simulink model "launchpad"  (R2014a)
settings: Solver=FixedStepDiscrete  StartTime=0.0  StopTime=10  FixedStep=0.1  RelTol=1e-3
PreLoadFcn:
  | use_hardware = 0;
  | hardware_variant = Simulink.Variant('use_hardware == 1');
  | software_variant = Simulink.Variant('use_hardware == 0');
undefined symbols (not defined in the file or in its folder): sigbuilder_block
libraries: launchpad_lib x5, simulink x1
settings Model: Creator=bas  LastModifiedBy=peselnikmg
settings OptimizationCC: InlineParams=on  UseFloatMulNetSlope=on  UseSpecifiedMinMax=on  InlineInvariantSignals=on  ExpressionDepthLimit=2147483647  ZeroExternalMemoryAtStartup=off  ZeroInternalMemoryAtStartup=off  NoFixptDivByZeroProtection=on  EfficientFloat2IntCast=on  OptimizeModelRefInitCode=on  LifeSpan=Inf
settings DebuggingCC: MergeDetectMultiDrivingBlocksExec=error  InheritedTsInSrcMsg=none  StateNameClashWarn=warning  StrictBusMsg=ErrorOnBusTreatedAsVector
settings HardwareCC: ProdBitPerInt=16  ProdBitPerPointer=16  ProdIntDivRoundTo=Zero  ProdEndianess=LittleEndian  ProdWordSize=16  ProdHWDeviceType=Texas Instruments->MSP430
settings RTWCC: SystemTargetFile=launchpad.tlc  TemplateMakefile=launchpad_tmf  Description=TI LaunchPad  GenerateReport=on  ProcessScript=launchpad_make_rtw_hook  IncludeHyperlinkInReport=on  LaunchReport=on  GenerateTraceInfo=on  GenerateTraceReport=on  GenerateTraceReportSl=on  GenerateTraceReportSf=on  GenerateTraceReportEml=on  GenerateCodeMetricsReport=on
settings CodeAppCC: IgnoreCustomStorageClasses=off  CustomSymbolStrType=$N$R$M  InternalIdentifier=Classic
settings STFCustomTargetCC: ConcurrentExecutionCompliant=off  IncludeMdlTerminateFcn=off  GeneratePreprocessorConditionals=Use local settings  CombineOutputUpdateFcns=on  CombineSignalStateStructs=on  SuppressErrorStatus=on  ERTCustomFileBanners=on  SupportNonFinite=off  SupportContinuousTime=off  SupportNonInlinedSFcns=off  MATLABClassNameForMDSCustomization=Simulink.SoftwareTarget.ERTCustomization  GRTInterface=off  SystemTargetFile=launchpad.tlc
settings ERTTargetCC: GenerateSampleERTMain=off  IncludeMdlTerminateFcn=off  CombineSignalStateStructs=on  SuppressErrorStatus=on  SupportNonFinite=off  ExtModeMexFile=noextcomm  ERTCustomFileTemplate=launchpad_srmain.tlc  ConvertIfToSwitch=on  SuppressUnreachableDefaultCases=on

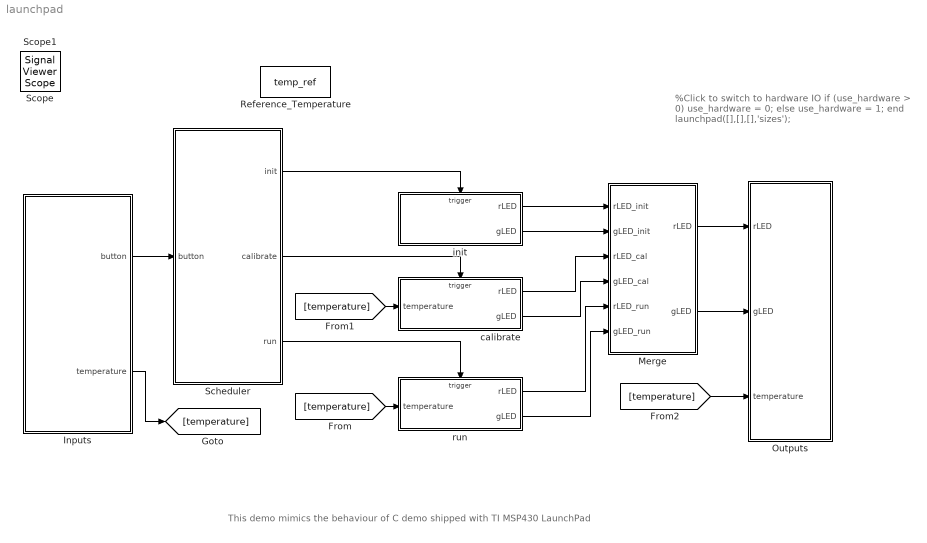
== system launchpad ==
  note: This demo mimics the behaviour of C demo shipped with TI MSP430 LaunchPad
  note: %Click to switch to hardware IO
      | if (use_hardware > 0)
      |     use_hardware = 0;
      | else
      |     use_hardware = 1;
      | end
      | launchpad([],[],[],'sizes');
  Inputs : Subsystem  Variant=on
  Merge : Subsystem
  Outputs : Subsystem  Variant=on
  Reference_Temperature : DataStoreMemory  DataStoreName=temp_ref  ReadBeforeWriteMsg=warning  WriteAfterWriteMsg=warning  WriteAfterReadMsg=warning  OutDataTypeStr=int8
  Scheduler : Subsystem
  calibrate : Subsystem
  init : Subsystem
  run : Subsystem
  Scope : SignalViewerScope  IOType=viewer  NumInputPorts=3  RefreshTime=0.035000
      settings: TimeRange=10  YMin=0~0~0  YMax=1~120~1
  Scope1 : SignalViewerScope  IOType=viewer  RefreshTime=0.035000
  wires:
  Scheduler/2(calibrate) -> calibrate/Trigger
  Scheduler/3(run) -> run/Trigger
  Inputs/1(button) -> Scheduler/1(button)
  Merge/1(rLED) -> Outputs/1(rLED)
  Merge/2(gLED) -> Outputs/2(gLED)
  calibrate/1(rLED) -> Merge/3(rLED_cal)
  calibrate/2(gLED) -> Merge/4(gLED_cal)
  run/1(rLED) -> Merge/5(rLED_run)
  run/2(gLED) -> Merge/6(gLED_run)
  init/1(rLED) -> Merge/1(rLED_init)
  init/2(gLED) -> Merge/2(gLED_init)
  Inputs/2(temperature) -> [temperature]
  [temperature] -> run/1(temperature)
  [temperature] -> calibrate/1(temperature)
  [temperature] -> Outputs/3(temperature)
  Scheduler/1(init) -> init/Trigger

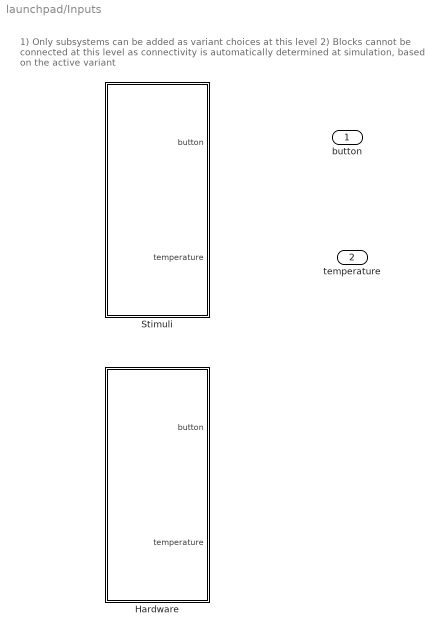
== system launchpad/Inputs ==
  note: 1) Only subsystems can be added as variant choices at this level
      | 2) Blocks cannot be connected at this level as connectivity is
      | automatically determined at simulation, based on the active variant
  Hardware : Subsystem  VariantControl=hardware_variant
  Stimuli : Subsystem  VariantControl=software_variant
  button : Outport
  temperature : Outport  Port=2

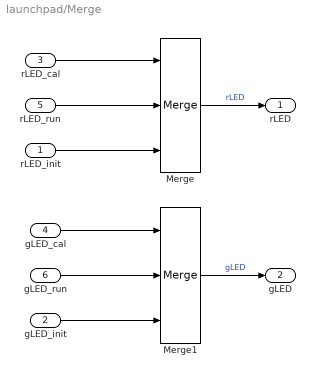
== system launchpad/Merge ==
  rLED_init : Inport
  gLED_init : Inport  Port=2
  rLED_cal : Inport  Port=3
  gLED_cal : Inport  Port=4
  rLED_run : Inport  Port=5
  gLED_run : Inport  Port=6
  Merge : Merge  Inputs=3  InitialOutput=0
  Merge1 : Merge  Inputs=3  InitialOutput=0
  rLED : Outport
  gLED : Outport  Port=2
  wires:
  rLED_cal/1 -> Merge/1
  Merge/1 -> rLED/1  "rLED"
  rLED_run/1 -> Merge/2
  gLED_cal/1 -> Merge1/1
  Merge1/1 -> gLED/1  "gLED"
  gLED_run/1 -> Merge1/2
  rLED_init/1 -> Merge/3
  gLED_init/1 -> Merge1/3

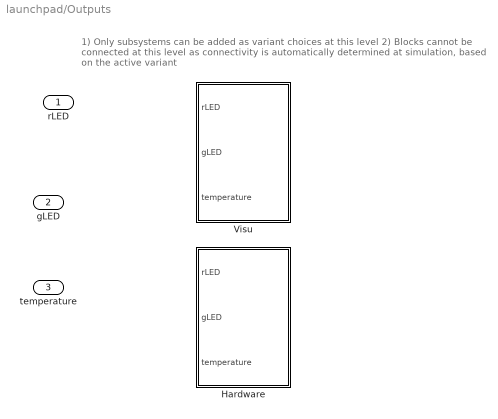
== system launchpad/Outputs ==
  note: 1) Only subsystems can be added as variant choices at this level
      | 2) Blocks cannot be connected at this level as connectivity is
      | automatically determined at simulation, based on the active variant
  rLED : Inport
  gLED : Inport  Port=2
  temperature : Inport  Port=3
  Hardware : Subsystem  VariantControl=hardware_variant
  Visu : Subsystem  VariantControl=software_variant

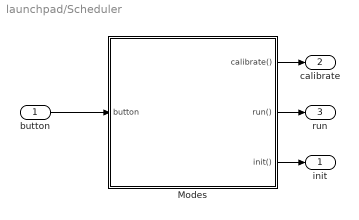
== system launchpad/Scheduler ==
  button : Inport
  Modes : Stateflow chart  TreatAsAtomicUnit=on
  init : Outport
  calibrate : Outport  Port=2
  run : Outport  Port=3
  wires:
  Modes/1(calibrate()) -> calibrate/1
  Modes/2(run()) -> run/1
  button/1 -> Modes/1(button)
  Modes/3(init()) -> init/1

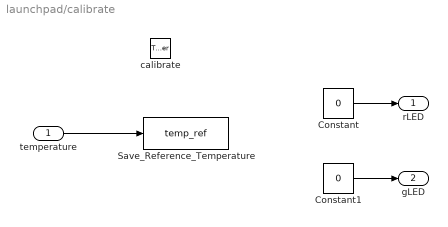
== system launchpad/calibrate ==
  temperature : Inport
  calibrate : TriggerPort  TriggerType=function-call  PortDimensions=1
  Constant : Constant  Value=0  OutDataTypeStr=uint8
  Constant1 : Constant  Value=0  OutDataTypeStr=uint8
  Save_Reference_Temperature : DataStoreWrite  DataStoreName=temp_ref
  rLED : Outport  InitialOutput=0
  gLED : Outport  Port=2  InitialOutput=0
  wires:
  Constant/1 -> rLED/1
  Constant1/1 -> gLED/1
  temperature/1 -> Save_Reference_Temperature/1

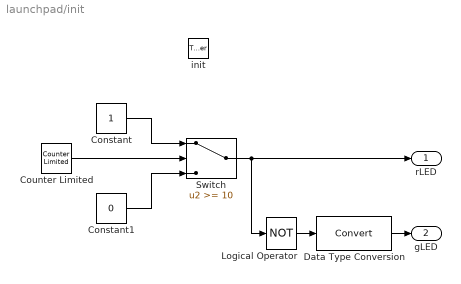
== system launchpad/init ==
  init : TriggerPort  TriggerType=function-call  PortDimensions=1
  Constant : Constant  OutDataTypeStr=uint8
  Constant1 : Constant  Value=0  OutDataTypeStr=uint8
  Counter Limited : simulink/Sources/Counter Limited  uplimit=19  tsamp=-1
      settings: AttributesFormatString=Limit=%<uplimit>
  Data Type Conversion : DataTypeConversion
  Logical Operator : Logic  Operator=NOT  AllPortsSameDT=off  OutDataTypeStr=boolean
  Switch : Switch  Threshold=10
      settings: AttributesFormatString=Threshold=%<Threshold>
  rLED : Outport
  gLED : Outport  Port=2
  wires:
  Switch/1 -> rLED/1, Logical Operator/1
  Counter Limited/1 -> Switch/2
  Constant1/1 -> Switch/3
  Constant/1 -> Switch/1
  Logical Operator/1 -> Data Type Conversion/1
  Data Type Conversion/1 -> gLED/1

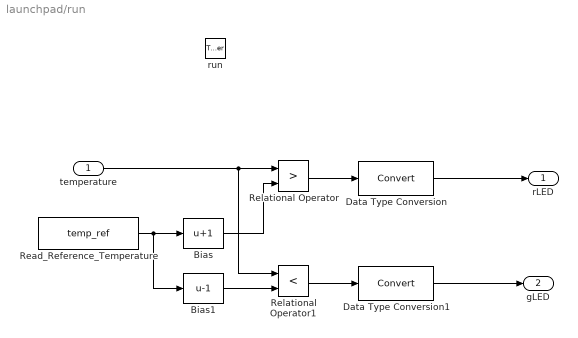
== system launchpad/run ==
  temperature : Inport
  run : TriggerPort  TriggerType=function-call  PortDimensions=1
  Bias : Bias  Bias=1
  Bias1 : Bias  Bias=-1
  Data Type Conversion : DataTypeConversion
  Data Type Conversion1 : DataTypeConversion
  Read_Reference_Temperature : DataStoreRead  DataStoreName=temp_ref
  Relational Operator : RelationalOperator  Operator=>  OutDataTypeStr=boolean
  Relational Operator1 : RelationalOperator  Operator=<  OutDataTypeStr=boolean
  rLED : Outport
  gLED : Outport  Port=2
  wires:
  temperature/1 -> Relational Operator/1, Relational Operator1/1
  Read_Reference_Temperature/1 -> Bias/1, Bias1/1
  Relational Operator/1 -> Data Type Conversion/1
  Bias/1 -> Relational Operator/2
  Bias1/1 -> Relational Operator1/2
  Relational Operator1/1 -> Data Type Conversion1/1
  Data Type Conversion1/1 -> gLED/1
  Data Type Conversion/1 -> rLED/1

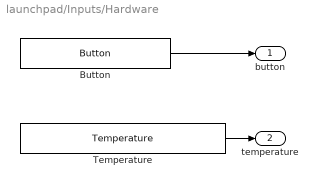
== system launchpad/Inputs/Hardware ==
  Button : launchpad_lib/Button
  Temperature : launchpad_lib/Temperature  SParameter1=Celsius
      settings: AttributesFormatString=%<SParameter1>
  button : Outport  OutDataTypeStr=uint8
  temperature : Outport  Port=2  OutDataTypeStr=int8
  wires:
  Temperature/1 -> temperature/1
  Button/1 -> button/1

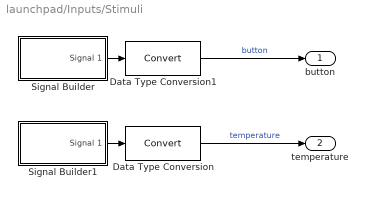
== system launchpad/Inputs/Stimuli ==
  Data Type Conversion : DataTypeConversion
  Data Type Conversion1 : DataTypeConversion
  Signal Builder : Subsystem  Tag=STV Subsys  LoadFcn=sigbuilder_block('load');  StartFcn=sigbuilder_block('start');  StopFcn=sigbuilder_block('stop');  ClipboardFcn=sigbuilder_block('clipboard');  mask(Sigbuilder block){}
      mask help: Simulink:masks:SigbuilderBlock_MD
      mask init:
      | if ~strcmp(get_param(bdroot(gcbh),'SimulationStatus'),'stopped') tuvar = sigbuilder_block('maskInit'); end
      settings: CopyFcn=sigbuilder_block('copy');  DeleteFcn=sigbuilder_block('delete');  ModelCloseFcn=sigbuilder_block('modelClose');  PreSaveFcn=sigbuilder_block('preSave');  PauseFcn=sigbuilder_block('pause');  ContinueFcn=sigbuilder_block('continue');  NameChangeFcn=sigbuilder_block('namechange');  OpenFcn=sigbuilder_block('open',[99 153 550.5 399.75 ]);  CloseFcn=sigbuilder_block('close');
      mask Display: plot(0, 0, 100, 100,[2, 2, 32, 32, 2], [68, 8, 8, 68, 68],[32, 2], [38, 38], [32, 19, 2],[53, 60, 44], [32, 17, 17, 2],[16, 16, 31, 31]);txt = getActiveGroup(gcbh);text(2, 100, txt,'verticalAlignment', 'top');
  Signal Builder1 : Subsystem  Tag=STV Subsys  LoadFcn=sigbuilder_block('load');  StartFcn=sigbuilder_block('start');  StopFcn=sigbuilder_block('stop');  ClipboardFcn=sigbuilder_block('clipboard');  mask(Sigbuilder block){}
      mask help: Simulink:masks:SigbuilderBlock_MD
      mask init:
      | if ~strcmp(get_param(bdroot(gcbh),'SimulationStatus'),'stopped') tuvar = sigbuilder_block('maskInit'); end
      settings: CopyFcn=sigbuilder_block('copy');  DeleteFcn=sigbuilder_block('delete');  ModelCloseFcn=sigbuilder_block('modelClose');  PreSaveFcn=sigbuilder_block('preSave');  PauseFcn=sigbuilder_block('pause');  ContinueFcn=sigbuilder_block('continue');  NameChangeFcn=sigbuilder_block('namechange');  OpenFcn=sigbuilder_block('open',[437.25 199.5 550.5 399.75 ]);  CloseFcn=sigbuilder_block('close');
      mask Display: plot(0, 0, 100, 100,[2, 2, 32, 32, 2], [68, 8, 8, 68, 68],[32, 2], [38, 38], [32, 19, 2],[53, 60, 44], [32, 17, 17, 2],[16, 16, 31, 31]);txt = getActiveGroup(gcbh);text(2, 100, txt,'verticalAlignment', 'top');
  button : Outport  OutDataTypeStr=uint8
  temperature : Outport  Port=2  OutDataTypeStr=int8
  wires:
  Data Type Conversion1/1 -> button/1  "button"
  Data Type Conversion/1 -> temperature/1  "temperature"
  Signal Builder1/1(Signal 1) -> Data Type Conversion/1
  Signal Builder/1(Signal 1) -> Data Type Conversion1/1

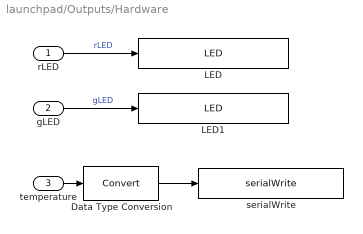
== system launchpad/Outputs/Hardware ==
  rLED : Inport
  gLED : Inport  Port=2
  temperature : Inport  Port=3
  Data Type Conversion : DataTypeConversion
  LED : launchpad_lib/LED  SParameter1=Red
      settings: AttributesFormatString=LED: %<SParameter1>
  LED1 : launchpad_lib/LED  SParameter1=Green
      settings: AttributesFormatString=LED: %<SParameter1>
  serialWrite : launchpad_lib/serialWrite
  wires:
  rLED/1 -> LED/1  "rLED"
  gLED/1 -> LED1/1  "gLED"
  temperature/1 -> Data Type Conversion/1
  Data Type Conversion/1 -> serialWrite/1

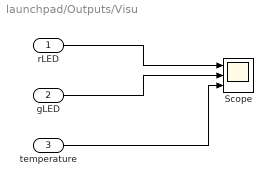
== system launchpad/Outputs/Visu ==
  rLED : Inport
  gLED : Inport  Port=2
  temperature : Inport  Port=3
  Scope : Scope  NumInputPorts=3
      settings: TimeRange=10  YMin=0~0~0  YMax=1~1~120
  wires:
  rLED/1 -> Scope/1
  gLED/1 -> Scope/2
  temperature/1 -> Scope/3

== system launchpad/Inputs/Stimuli/Signal Builder ==
  Demux : Demux  Tag=STV Demux  Outputs=1
  FromWs : FromWorkspace  Tag=STV FromWs  VariableName=tuvar  SampleTime=0
      SigBuilderData=|
      | common.afterFinalStr = 'Extrapolate'
      | common.sampleTime = 0
      | dataSet.timeRange = [0 10]
      | dataSet.name = 'Group 1'
      | sbobj.Groups.Name = 'Group 1'
      | sbobj.Groups.Signals.Name = 'Signal 1'
      | sbobj.Groups.Signals.XData = [0 3 3 3.1 3.1 7 7 7.1 7.1 10]
      | sbobj.Groups.Signals.YData = [0 0 1 1 0 0 1 1 0 0]
  Signal 1 : Outport  Tag=STV Outport
  wires:
  FromWs/1 -> Demux/1
  Demux/1 -> Signal 1/1

== system launchpad/Inputs/Stimuli/Signal Builder1 ==
  Demux : Demux  Tag=STV Demux  Outputs=1
  FromWs : FromWorkspace  Tag=STV FromWs  VariableName=tuvar  SampleTime=0
      SigBuilderData=|
      | common.afterFinalStr = 'Extrapolate'
      | common.sampleTime = 0
      | dataSet.timeRange = [0 10]
      | dataSet.name = 'Group 1'
      | sbobj.Groups.Name = 'Group 1'
      | sbobj.Groups.Signals.Name = 'Signal 1'
      | sbobj.Groups.Signals.XData = [0 5 6.28 10]
      | sbobj.Groups.Signals.YData = [0 110 35.5 0]
  Signal 1 : Outport  Tag=STV Outport
  wires:
  Demux/1 -> Signal 1/1
  FromWs/1 -> Demux/1

== stateflow chart launchpad/Scheduler/Modes ==
  state Init
    du:init;
  state Run
    state execute
      en:run;
    execute -> execute : after(10,tick)
  state Calibrate
    en:calibrate;
  (default) -> Init
  Init -> Calibrate : [button > 0]
  Calibrate -> Run
  Run -> Calibrate : [button > 0]
  data: button input
  events: calibrate output FUNCTION_CALL_EVENT; run output FUNCTION_CALL_EVENT; init output FUNCTION_CALL_EVENT
